simulink model "temperaturetank"  (R2024b)
settings: Solver=VariableStepAuto  StartTime=0.0  StopTime=10.0  RelTol=1e-3
settings Model: Creator=Krishna K S  LastModifiedBy=Krishna K S

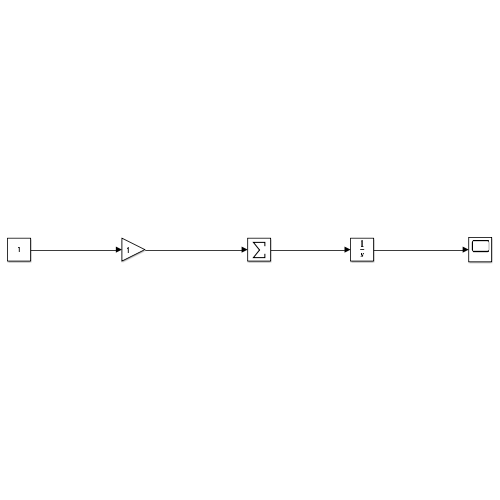
[thumbnail: Simulink's stored preview of the top-level diagram]
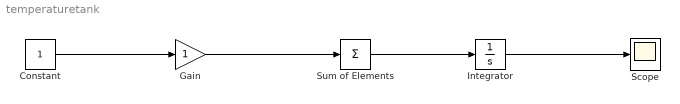
== system temperaturetank ==
  Constant : Constant
  Gain : Gain
  Integrator : Integrator
  Scope : Scope
  Sum of Elements : Sum  Inputs=+
  wires:
  Constant/1 -> Gain/1
  Gain/1 -> Sum of Elements/1
  Sum of Elements/1 -> Integrator/1
  Integrator/1 -> Scope/1
